simulink model "single_battery_BMS_OCV"  (R2024b)
settings: Solver=VariableStepAuto  StartTime=0.0  StopTime=10.0  RelTol=1e-3
libraries: simulink x3
settings Model: Creator=nirmithpuneet  LastModifiedBy=nirmithpuneet

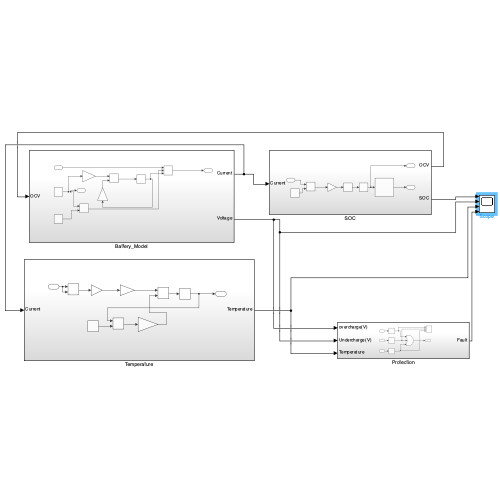
[thumbnail: Simulink's stored preview of the top-level diagram]
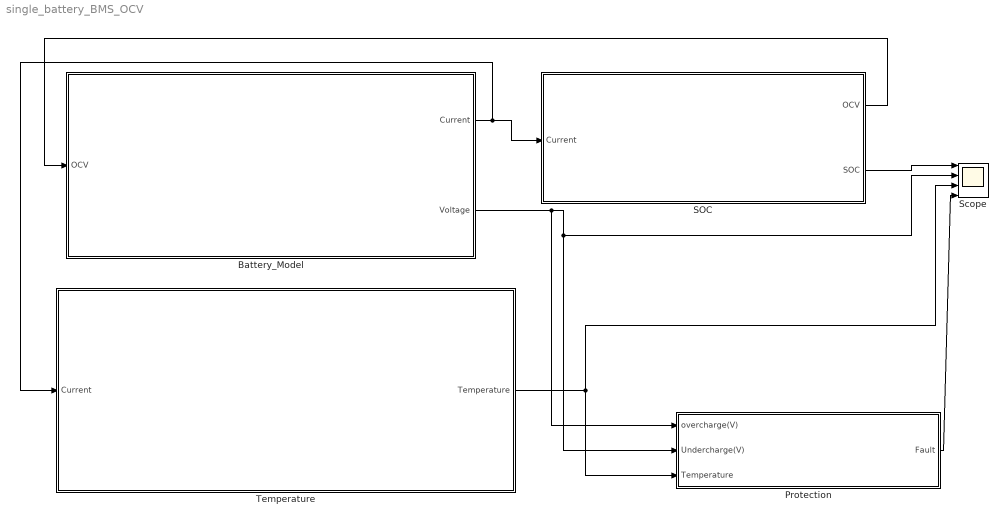
== system single_battery_BMS_OCV ==
  Battery_Model : Subsystem
  Protection : Subsystem
  SOC : Subsystem
  Scope : Scope  NumInputPorts=4
  Temperature : Subsystem
  wires:
  Battery_Model/1(Current) -> Temperature/1(Current), SOC/1(Current)
  SOC/2(SOC) -> Scope/1
  Battery_Model/2(" Voltage") -> Protection/1(overcharge(V)), Protection/2(Undercharge(V)), Scope/2
  Temperature/1(Temperature) -> Protection/3(Temperature), Scope/3
  SOC/1(OCV) -> Battery_Model/1(OCV)
  Protection/1(Fault) -> Scope/4

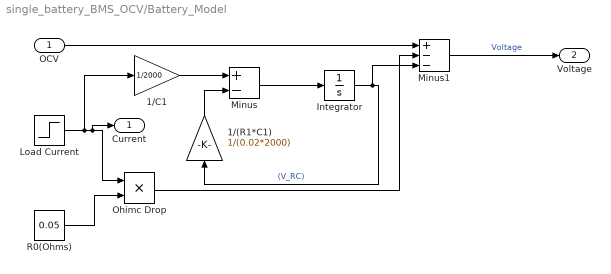
== system single_battery_BMS_OCV/Battery_Model ==
  OCV : Inport
  1/(R1*C1) : Gain  Gain=1/(0.02*2000)
  1/C1 : Gain  Gain=1/2000
  Integrator : Integrator
  Load Current : Step  After=5  SampleTime=0
  Minus : Sum  Inputs=+-
  Minus1 : Sum  Inputs=+--
  Ohimc Drop : Product
  R0(Ohms) : Constant  Value=0.05
  Current : Outport
  " Voltage" : Outport  Port=2
  wires:
  Ohimc Drop/1 -> Minus1/2
  1/(R1*C1)/1 -> Minus/2
  Minus/1 -> Integrator/1
  Load Current/1 -> 1/C1/1, Current/1, Ohimc Drop/1
  Minus1/1 -> " Voltage"/1  "Voltage"
  1/C1/1 -> Minus/1
  OCV/1 -> Minus1/1
  R0(Ohms)/1 -> Ohimc Drop/2
  Integrator/1 -> Minus1/3, 1/(R1*C1)/1  "(V_RC)"

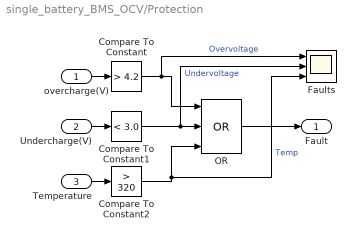
== system single_battery_BMS_OCV/Protection ==
  overcharge(V) : Inport
  Undercharge(V) : Inport  Port=2
  Temperature : Inport  Port=3
  Compare To Constant : simulink/Logic and Bit Operations/Compare To Constant  relop=>  const=4.2  OutDataTypeStr=boolean
  Compare To Constant1 : simulink/Logic and Bit Operations/Compare To Constant  relop=<  const=3.0  OutDataTypeStr=boolean
  Compare To Constant2 : simulink/Logic and Bit Operations/Compare To Constant  relop=>  const=320  OutDataTypeStr=boolean
  Faults : Scope  NumInputPorts=3
  OR : Logic  Operator=OR  Inputs=3  IconShape=distinctive  AllPortsSameDT=off  OutDataTypeStr=boolean
  Fault : Outport
  wires:
  Temperature/1 -> Compare To Constant2/1
  Compare To Constant/1 -> Faults/1, OR/1  "Overvoltage"
  Undercharge(V)/1 -> Compare To Constant1/1
  overcharge(V)/1 -> Compare To Constant/1
  Compare To Constant1/1 -> Faults/2, OR/2  "Undervoltage"
  Compare To Constant2/1 -> Faults/3, OR/3  "Temp"
  OR/1 -> Fault/1

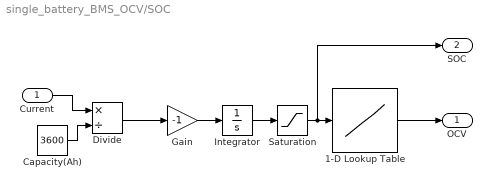
== system single_battery_BMS_OCV/SOC ==
  Current : Inport
  1-D Lookup Table : Lookup_n-D  NumberOfTableDimensions=1  BreakpointsForDimension1=[0 0.2 0.5 0.8 1]  Table=[3.0 3.3 3.6 3.9 4.2]  ExtrapMethod=Clip  InternalRulePriority=Speed  RndMeth=Simplest
  Capacity(Ah) : Constant  Value=3600
  Divide : Product  Inputs=*/
  Gain : Gain  Gain=-1
  Integrator : Integrator  InitialCondition=1
  Saturation : Saturate  UpperLimit=1  LowerLimit=0
  OCV : Outport
  SOC : Outport  Port=2
  wires:
  Current/1 -> Divide/1
  Capacity(Ah)/1 -> Divide/2
  Integrator/1 -> Saturation/1
  Gain/1 -> Integrator/1
  Divide/1 -> Gain/1
  Saturation/1 -> SOC/1, 1-D Lookup Table/1
  1-D Lookup Table/1 -> OCV/1

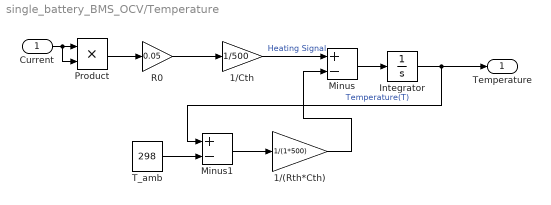
== system single_battery_BMS_OCV/Temperature ==
  Current : Inport
  1/(Rth*Cth) : Gain  Gain=1/(1*500)
  1/Cth : Gain  Gain=1/500
  Integrator : Integrator  InitialCondition=298
  Minus : Sum  Inputs=+-
  Minus1 : Sum  Inputs=+-
  Product : Product
  R0 : Gain  Gain=0.05
  T_amb : Constant  Value=298
  Temperature : Outport
  wires:
  Product/1 -> R0/1
  R0/1 -> 1/Cth/1
  Minus/1 -> Integrator/1
  Minus1/1 -> 1/(Rth*Cth)/1
  Current/1 -> Product/2, Product/1
  T_amb/1 -> Minus1/2
  1/Cth/1 -> Minus/1  "Heating Signal"
  Integrator/1 -> Temperature/1, Minus1/1  "Temperature(T)"
  1/(Rth*Cth)/1 -> Minus/2
